simulink model "test_model_replacement"  (R2020a)
settings: Solver=FixedStepDiscrete  StartTime=0.0  StopTime=10.0  FixedStep=0.01  RelTol=1e-3
settings Model: sldv_blockreplacement_configurable_lib=test_model_rt_lib  Creator=1014721  LastModifiedBy=1014721
settings OptimizationCC: DefaultParameterBehavior=Inlined  EnhancedBackFolding=on  PassReuseOutputArgsAs=Individual arguments  ZeroExternalMemoryAtStartup=off  ZeroInternalMemoryAtStartup=off  OptimizeBlockOrder=speed  DifferentSizesBufferReuse=on  OptimizationCustomize=off  EfficientTunableParamExpr=on
settings DebuggingCC: SaveWithParameterizedLinksMsg=none  ParameterTunabilityLossMsg=error
settings SFSimCC: MATLABDynamicMemAlloc=off
settings RTWCC: SystemTargetFile=ert.tlc  GenCodeOnly=on  TemplateMakefile=ert_default_tmf  GenerateReport=on  LaunchReport=on
settings CodeAppCC: ForceParamTrailComments=on  IgnoreCustomStorageClasses=off  OperatorAnnotations=on  SimulinkDataObjDesc=on  SFDataObjDesc=on  InsertBlockDesc=on
settings ERTTargetCC: TargetLangStandard=C99 (ISO)  GenerateSampleERTMain=on  InlinedParameterPlacement=NonHierarchical  ERTCustomFileTemplate=example_file_process.tlc
settings ConfigComp: DVTestSuiteOptimization=Auto  DVDetectOutOfBounds=on

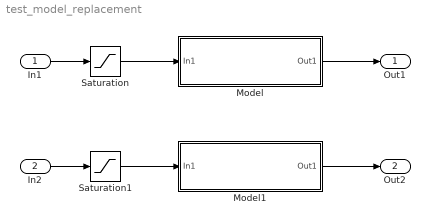
== system test_model_replacement ==
  In1 : Inport
  In2 : Inport  Port=2
  Model : Subsystem  mask(Sldv ModelReference(Model name:test_ref_model) Replacement){judge_val=10, output_val=1, SimulationMode=Normal, ModelName=test_ref_model, ParameterArgumentNames=judge_val,output_val, ParameterArgumentValuesAsString=judge_val,output_val}
      mask prompts: SimulationMode "Simulink:blkprm_prompts:ModelRefSimulationMode"
      mask help: Replacement for the Model Reference block that references the model test_ref_model. If Model arguments are specified on the Model Reference block, then they will appear in the mask parameters.
      mask TypeOptions SimulationMode: SimulationMode
      mask DialogControl SimulationMode Prompt: シミュレーション モード:
  Model1 : Subsystem  mask(Sldv ModelReference(Model name:test_ref_model) Replacement){judge_val=10, output_val=1, SimulationMode=Normal, ModelName=test_ref_model, ParameterArgumentNames=judge_val,output_val, ParameterArgumentValuesAsString=judge_val,output_val}
      mask prompts: SimulationMode "Simulink:blkprm_prompts:ModelRefSimulationMode"
      mask help: Replacement for the Model Reference block that references the model test_ref_model. If Model arguments are specified on the Model Reference block, then they will appear in the mask parameters.
      mask TypeOptions SimulationMode: SimulationMode
      mask DialogControl SimulationMode Prompt: シミュレーション モード:
  Saturation : Saturate  UpperLimit=20  LowerLimit=-20
      settings: AttributesFormatString=|
      | 上限：%<UpperLimit>
      | 下限：%<LowerLimit>
  Saturation1 : Saturate  UpperLimit=5  LowerLimit=-5
      settings: AttributesFormatString=|
      | 上限：%<UpperLimit>
      | 下限：%<LowerLimit>
  Out1 : Outport
  Out2 : Outport  Port=2
  wires:
  In1/1 -> Saturation/1
  Model/1(Out1) -> Out1/1
  Saturation/1 -> Model/1(In1)
  Saturation1/1 -> Model1/1(In1)
  In2/1 -> Saturation1/1
  Model1/1(Out1) -> Out2/1

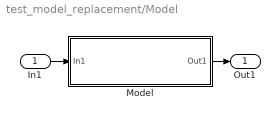
== system test_model_replacement/Model ==
  In1 : Inport
  Model : Subsystem  TreatAsAtomicUnit=on
  Out1 : Outport  OutDataTypeStr=int32  PortDimensions=1  SampleTime=[0.01,0]
  wires:
  Model/1(Out1) -> Out1/1
  In1/1 -> Model/1(In1)

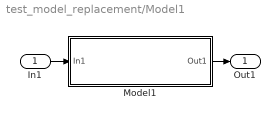
== system test_model_replacement/Model1 ==
  In1 : Inport
  Model1 : Subsystem  TreatAsAtomicUnit=on
  Out1 : Outport  OutDataTypeStr=int32  PortDimensions=1  SampleTime=[0.01,0]
  wires:
  Model1/1(Out1) -> Out1/1
  In1/1 -> Model1/1(In1)

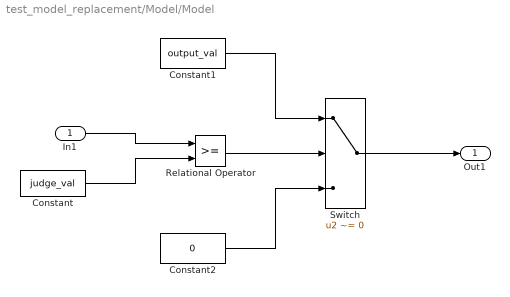
== system test_model_replacement/Model/Model ==
  In1 : Inport  OutDataTypeStr=int32  PortDimensions=1  SampleTime=[0.01,0]
  Constant : Constant  Value=judge_val  OutDataTypeStr=int32
  Constant1 : Constant  Value=output_val  OutDataTypeStr=int32
  Constant2 : Constant  Value=0  OutDataTypeStr=int32
  Relational Operator : RelationalOperator  OutDataTypeStr=boolean  RndMeth=Simplest
  Switch : Switch  Criteria=u2 ~= 0
  Out1 : Outport  OutDataTypeStr=int32
  wires:
  Constant1/1 -> Switch/1
  Constant2/1 -> Switch/3
  Switch/1 -> Out1/1
  Relational Operator/1 -> Switch/2
  Constant/1 -> Relational Operator/2
  In1/1 -> Relational Operator/1

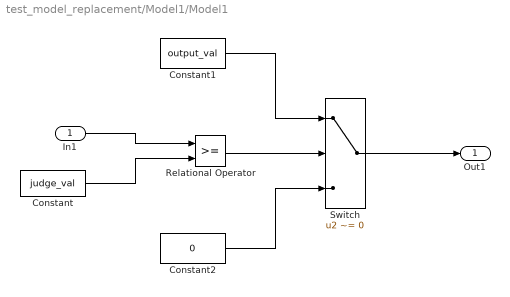
== system test_model_replacement/Model1/Model1 ==
  In1 : Inport  OutDataTypeStr=int32  PortDimensions=1  SampleTime=[0.01,0]
  Constant : Constant  Value=judge_val  OutDataTypeStr=int32
  Constant1 : Constant  Value=output_val  OutDataTypeStr=int32
  Constant2 : Constant  Value=0  OutDataTypeStr=int32
  Relational Operator : RelationalOperator  OutDataTypeStr=boolean  RndMeth=Simplest
  Switch : Switch  Criteria=u2 ~= 0
  Out1 : Outport  OutDataTypeStr=int32
  wires:
  Constant1/1 -> Switch/1
  Constant2/1 -> Switch/3
  Switch/1 -> Out1/1
  Relational Operator/1 -> Switch/2
  Constant/1 -> Relational Operator/2
  In1/1 -> Relational Operator/1
